simulink model "r1"  (Simulink 8.6)
settings: Solver=FixedStepDiscrete  StartTime=0.0  StopTime=10.0  FixedStep=1  RelTol=1e-3
undefined symbols (not defined in the file): sldvsubsys
libraries: sldvlib x10, simulink x1
settings Model: Creator=elliocm  LastModifiedBy=mike
settings DataIOCC: SignalLoggingSaveFormat=Dataset
settings DebuggingCC: IntegerOverflowMsg=none  FcnCallInpInsideContextMsg=EnableAllAsError  IntegerSaturationMsg=none
settings GRTTargetCC: CombineOutputUpdateFcns=on  GRTInterface=off
settings ConfigComp: DVMaxProcessTime=5000  DVMaxTestCaseSteps=500  DVTestSuiteOptimization=CombinedObjectives (Nonlinear Extended)  DVDetectActiveLogic=on

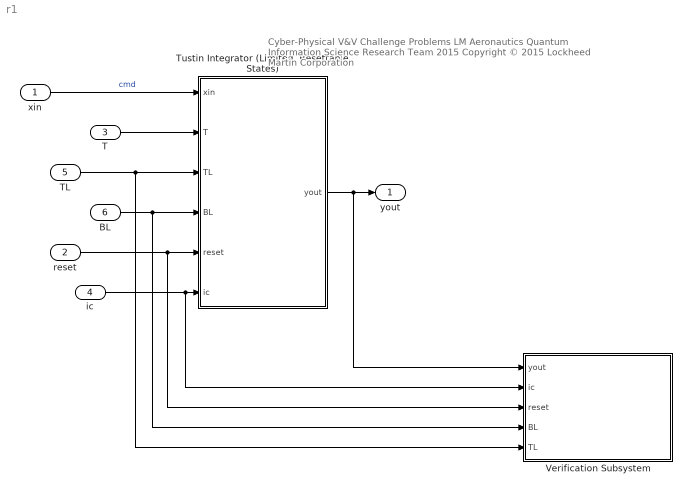
== system r1 ==
  note: Cyber-Physical V&V Challenge Problems
      | LM Aeronautics Quantum Information Science Research Team 2015
      | Copyright © 2015 Lockheed Martin Corporation
  xin : Inport  OutDataTypeStr=double
  reset : Inport  Port=2  OutDataTypeStr=boolean
  T : Inport  Port=3  OutDataTypeStr=double
  ic : Inport  Port=4  OutDataTypeStr=double
  TL : Inport  Port=5  OutDataTypeStr=double
  BL : Inport  Port=6  OutDataTypeStr=double
  "Tustin Integrator (Limited, Resettable, States)" : Subsystem
  Verification Subsystem : Subsystem  Tag=VerificationSubsystem  DisableCoverage=on  LoadFcn=sldvsubsys('check')  TreatAsAtomicUnit=on  SimViewingDevice=on  mask(VerificationSubsystem){}
      mask init:
      | sldvsubsys('maskInit');
      settings: CopyFcn=sldvsubsys('copy');  OpenFcn=open_system(gcb,'force');
      settings: PreSaveFcn=|
      | set_param(gcb,'SimViewingDevice','on');
      | sldvsubsys('check');
      mask Help: helpview(fullfile(docroot,'toolbox','sldv','sldv.map'),'verificationsubsystem')
      mask Display: image(imread('sldvicon_versubsys.png','BackGroundColor',[1 1 1]),'center');
  yout : Outport
  wires:
  BL/1 -> Verification Subsystem/4(BL), "Tustin Integrator (Limited, Resettable, States)"/4(BL)
  TL/1 -> Verification Subsystem/5(TL), "Tustin Integrator (Limited, Resettable, States)"/3(TL)
  reset/1 -> Verification Subsystem/3(reset), "Tustin Integrator (Limited, Resettable, States)"/5(reset)
  ic/1 -> Verification Subsystem/2(ic), "Tustin Integrator (Limited, Resettable, States)"/6(ic)
  "Tustin Integrator (Limited, Resettable, States)"/1(yout) -> Verification Subsystem/1(yout), yout/1
  T/1 -> "Tustin Integrator (Limited, Resettable, States)"/2(T)
  xin/1 -> "Tustin Integrator (Limited, Resettable, States)"/1(xin)  "cmd"

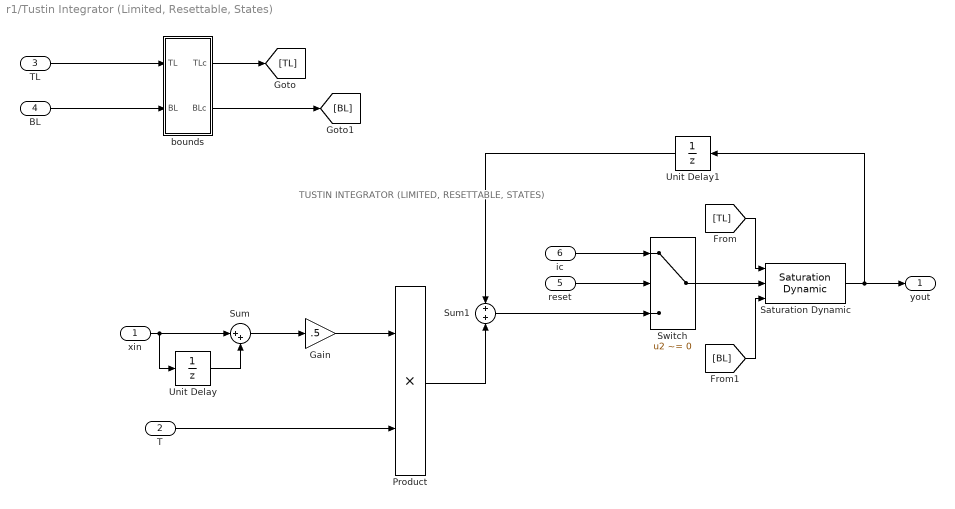
== system r1/Tustin Integrator (Limited, Resettable, States) ==
  note: TUSTIN INTEGRATOR (LIMITED, RESETTABLE, STATES)
  xin : Inport
  T : Inport  Port=2
  TL : Inport  Port=3
  BL : Inport  Port=4
  reset : Inport  Port=5
  ic : Inport  Port=6
  Gain : Gain  Gain=.5
  Product : Product  RndMeth=Zero
  Saturation Dynamic : simulink/Discontinuities/Saturation Dynamic  OutMin=[]  OutMax=[]  OutDataTypeStr=Inherit: Same as second input  OutDataType=fixdt(1, 16)  OutScaling=2^-10  DoSatur=off
  Sum : Sum  Inputs=|++
  Sum1 : Sum
  Switch : Switch  Criteria=u2 ~= 0  Threshold=0.5
  Unit Delay : UnitDelay  SampleTime=-1
  Unit Delay1 : UnitDelay  SampleTime=-1
  bounds : Subsystem
  yout : Outport
  wires:
  xin/1 -> Unit Delay/1, Sum/1
  Unit Delay/1 -> Sum/2
  Sum/1 -> Gain/1
  Gain/1 -> Product/1
  T/1 -> Product/2
  Product/1 -> Sum1/2
  Sum1/1 -> Switch/3
  reset/1 -> Switch/2
  ic/1 -> Switch/1
  Switch/1 -> Saturation Dynamic/2
  Saturation Dynamic/1 -> Unit Delay1/1, yout/1
  Unit Delay1/1 -> Sum1/1
  TL/1 -> bounds/1(TL)
  BL/1 -> bounds/2(BL)
  bounds/1(TLc) -> [TL]
  bounds/2(BLc) -> [BL]
  [TL] -> Saturation Dynamic/1
  [BL] -> Saturation Dynamic/3

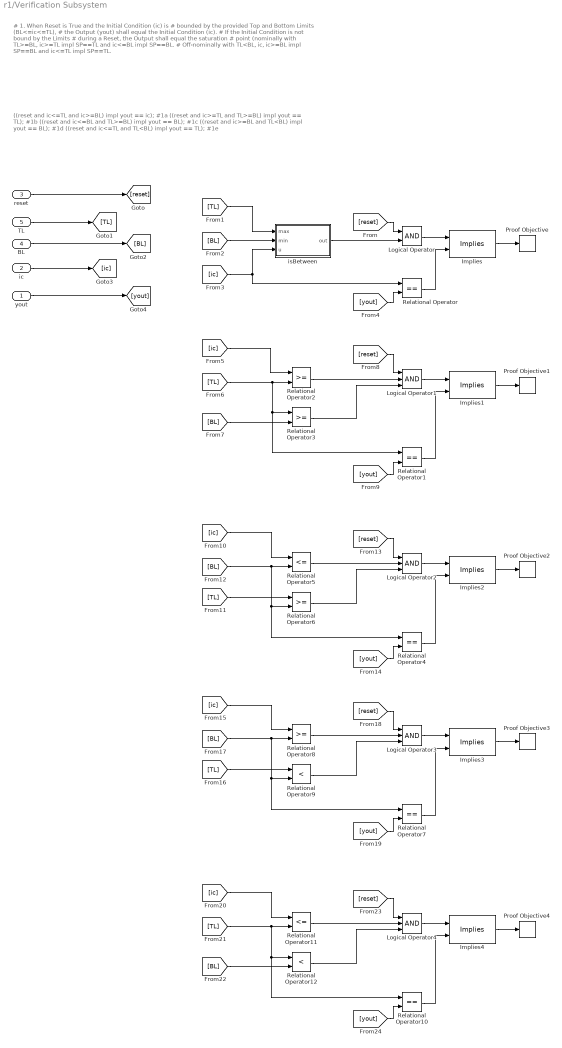
== system r1/Verification Subsystem ==
  note: # 1. When Reset is True and the Initial Condition (ic) is
      | # bounded by the provided Top and Bottom Limits (BL<=ic<=TL),
      | # the Output (yout) shall equal the Initial Condition (ic).
      | # If the Initial Condition is not bound by the Limits
      | # during a Reset, the Output shall equal the saturation
      | # point (nominally with TL>=BL, ic>=TL impl SP==TL and ic<=BL impl SP==BL.
      | # Off-nominally with TL<BL, ic, ic>=BL impl SP==BL and ic<=TL impl SP==TL.
  note: ((reset and ic<=TL and ic>=BL) impl yout == ic); #1a
      | ((reset and ic>=TL and TL>=BL) impl yout == TL); #1b
      | ((reset and ic<=BL and TL>=BL) impl yout == BL); #1c
      | ((reset and ic>=BL and TL<BL) impl yout == BL); #1d
      | ((reset and ic<=TL and TL<BL) impl yout == TL); #1e
  yout : Inport
  ic : Inport  Port=2
  reset : Inport  Port=3
  BL : Inport  Port=4
  TL : Inport  Port=5
  Implies{,1..4} (5 alike) : sldvlib/Verification Utilities/Implies
  Logical Operator : Logic  AllPortsSameDT=off  OutDataTypeStr=boolean
  Logical Operator{1..4} (4 alike) : Logic  Inputs=3  AllPortsSameDT=off  OutDataTypeStr=boolean
  Proof Objective{,1..4} (5 alike) : sldvlib/Objectives and Constraints/Proof Objective  enabled=on  customAVTBlockType=Proof Objective  intervals=true  dispValues=on  outEnabled=off  enableStopSim=off
      settings: AttributesFormatString=%<intervals>
  Relational Operator{,1,4,7,10} (5 alike) : RelationalOperator  Operator===  OutDataTypeStr=boolean
  Relational Operator11 : RelationalOperator  Operator=<=  OutDataTypeStr=boolean
  Relational Operator12 : RelationalOperator  Operator=<  OutDataTypeStr=boolean
  Relational Operator{2..3,6,8} (4 alike) : RelationalOperator  OutDataTypeStr=boolean
  Relational Operator5 : RelationalOperator  Operator=<=  OutDataTypeStr=boolean
  Relational Operator9 : RelationalOperator  Operator=<  OutDataTypeStr=boolean
  isBetween : Subsystem
  wires:
  BL/1 -> [BL]
  TL/1 -> [TL]
  ic/1 -> [ic]
  isBetween/1(out) -> Logical Operator/2
  Logical Operator/1 -> Implies/1
  yout/1 -> [yout]
  Relational Operator/1 -> Implies/2
  Implies/1 -> Proof Objective/1
  Relational Operator2/1 -> Logical Operator1/2
  reset/1 -> [reset]
  Logical Operator1/1 -> Implies1/1
  Relational Operator1/1 -> Implies1/2
  Implies1/1 -> Proof Objective1/1
  Relational Operator3/1 -> Logical Operator1/3
  [reset] -> Logical Operator/1
  [TL] -> isBetween/1(max)
  [BL] -> isBetween/2(min)
  [ic] -> Relational Operator/1, isBetween/3(u)
  [yout] -> Relational Operator/2
  [ic] -> Relational Operator2/1
  [TL] -> Relational Operator2/2, Relational Operator3/1, Relational Operator1/1
  [BL] -> Relational Operator3/2
  [reset] -> Logical Operator1/1
  [yout] -> Relational Operator1/2
  Relational Operator5/1 -> Logical Operator2/2
  Relational Operator4/1 -> Implies2/2
  Implies2/1 -> Proof Objective2/1
  Relational Operator6/1 -> Logical Operator2/3
  [ic] -> Relational Operator5/1
  [TL] -> Relational Operator6/1
  [BL] -> Relational Operator5/2, Relational Operator4/1, Relational Operator6/2
  [reset] -> Logical Operator2/1
  [yout] -> Relational Operator4/2
  Logical Operator2/1 -> Implies2/1
  Relational Operator8/1 -> Logical Operator3/2
  Relational Operator7/1 -> Implies3/2
  Relational Operator9/1 -> Logical Operator3/3
  [ic] -> Relational Operator8/1
  [TL] -> Relational Operator9/1
  [BL] -> Relational Operator8/2, Relational Operator7/1, Relational Operator9/2
  [reset] -> Logical Operator3/1
  [yout] -> Relational Operator7/2
  Logical Operator3/1 -> Implies3/1
  Implies3/1 -> Proof Objective3/1
  Relational Operator11/1 -> Logical Operator4/2
  Relational Operator10/1 -> Implies4/2
  Relational Operator12/1 -> Logical Operator4/3
  [ic] -> Relational Operator11/1
  [TL] -> Relational Operator11/2, Relational Operator10/1, Relational Operator12/1
  [BL] -> Relational Operator12/2
  [reset] -> Logical Operator4/1
  [yout] -> Relational Operator10/2
  Logical Operator4/1 -> Implies4/1
  Implies4/1 -> Proof Objective4/1

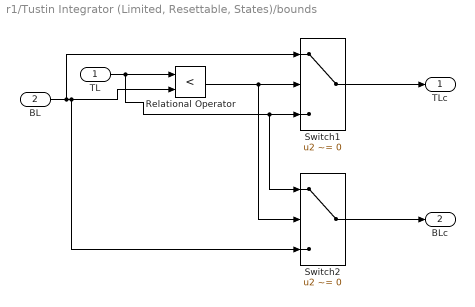
== system r1/Tustin Integrator (Limited, Resettable, States)/bounds ==
  TL : Inport
  BL : Inport  Port=2
  Relational Operator : RelationalOperator  Operator=<  OutDataTypeStr=boolean
  Switch1 : Switch  Criteria=u2 ~= 0  Threshold=0.5
  Switch2 : Switch  Criteria=u2 ~= 0  Threshold=0.5
  TLc : Outport
  BLc : Outport  Port=2
  wires:
  BL/1 -> Switch1/1, Switch2/3, Relational Operator/2
  TL/1 -> Switch2/1, Switch1/3, Relational Operator/1
  Relational Operator/1 -> Switch2/2, Switch1/2
  Switch1/1 -> TLc/1
  Switch2/1 -> BLc/1

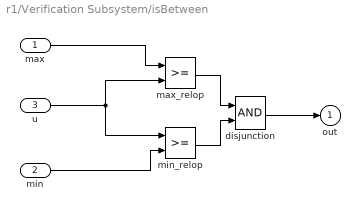
== system r1/Verification Subsystem/isBetween ==
  max : Inport
  min : Inport  Port=2
  u : Inport  Port=3
  disjunction : Logic  DisableCoverage=on
  max_relop : RelationalOperator  DisableCoverage=on
  min_relop : RelationalOperator  DisableCoverage=on
  out : Outport
  wires:
  disjunction/1 -> out/1
  max/1 -> max_relop/1
  min_relop/1 -> disjunction/2
  max_relop/1 -> disjunction/1
  min/1 -> min_relop/2
  u/1 -> max_relop/2, min_relop/1
